simulink model "PMSM_model"  (R2014b)
settings: Solver=ode45  StartTime=0.0  StopTime=10.0  RelTol=1e-3
settings Model: CovSFcnEnable=on  Creator=Lei  LastModifiedBy=Lei
settings DataIOCC: SignalLoggingSaveFormat=ModelDataLogs  SignalLoggingName=sigsOut
settings DebuggingCC: SaveWithParameterizedLinksMsg=none  UnderspecifiedInitializationDetection=Classic  MergeDetectMultiDrivingBlocksExec=none  SignalResolutionControl=TryResolveAllWithWarning  SolverPrmCheckMsg=none  MultiTaskDSMMsg=warning  MultiTaskCondExecSysMsg=none  FrameProcessingCompatibilityMsg=error  StrictBusMsg=None
settings HardwareCC: TargetUnknown=on
settings GRTTargetCC: CombineOutputUpdateFcns=off  GRTInterface=on

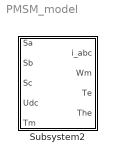
== system PMSM_model ==
  Subsystem2 : Subsystem

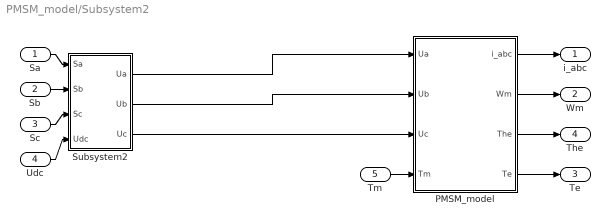
== system PMSM_model/Subsystem2 ==
  Sa : Inport
  Sb : Inport  Port=2
  Sc : Inport  Port=3
  Udc : Inport  Port=4
  Tm : Inport  Port=5
  PMSM_model : Subsystem  mask{Ld=0, Lq=0, R=0, Pn=0, flux=0, B=0, J=0}
      mask prompts: Ld "d-Inductances(Ld)"; Lq "q-Inductances(Lq)"; R "resistance(R)"; Pn "pole pairs(Pn)"; flux "Flux linkage(flux)"; B "viscous damping(B)"; J "Inertia(J)"
  Subsystem2 : Subsystem
  i_abc : Outport
  Wm : Outport  Port=2
  Te : Outport  Port=3
  The : Outport  Port=4
  wires:
  Sb/1 -> Subsystem2/2(Sb)
  Sc/1 -> Subsystem2/3(Sc)
  Udc/1 -> Subsystem2/4(Udc)
  Sa/1 -> Subsystem2/1(Sa)
  Subsystem2/1(Ua) -> PMSM_model/1(Ua)
  Subsystem2/2(Ub) -> PMSM_model/2(Ub)
  Subsystem2/3(Uc) -> PMSM_model/3(Uc)
  Tm/1 -> PMSM_model/4(Tm)
  PMSM_model/1(i_abc) -> i_abc/1
  PMSM_model/2(Wm) -> Wm/1
  PMSM_model/4(Te) -> Te/1
  PMSM_model/3(The) -> The/1

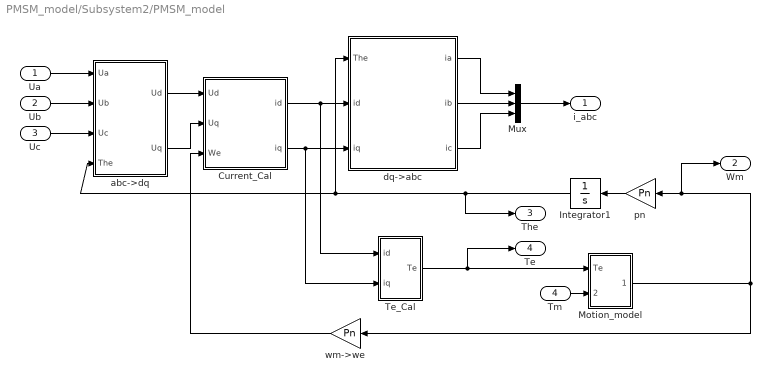
== system PMSM_model/Subsystem2/PMSM_model ==
  Ua : Inport
  Ub : Inport  Port=2
  Uc : Inport  Port=3
  Tm : Inport  Port=4
  Current_Cal : Subsystem
  Integrator1 : Integrator
  Motion_model : Subsystem
  Mux : Mux  Inputs=3
  Te_Cal : Subsystem
  abc->dq : Subsystem
  dq->abc : Subsystem
  pn : Gain  Gain=Pn  SaturateOnIntegerOverflow=on  OutDataTypeStr=Inherit: Same as input  ParamDataTypeStr=Inherit: Same as input
  wm->we : Gain  Gain=Pn  SaturateOnIntegerOverflow=on  OutDataTypeStr=Inherit: Same as input  ParamDataTypeStr=Inherit: Same as input
  i_abc : Outport
  Wm : Outport  Port=2
  The : Outport  Port=3
  Te : Outport  Port=4
  wires:
  Ua/1 -> abc->dq/1(Ua)
  abc->dq/1(Ud) -> Current_Cal/1(Ud)
  abc->dq/2(Uq) -> Current_Cal/2(Uq)
  Current_Cal/1(id) -> Te_Cal/1(id), dq->abc/2(id)
  Current_Cal/2(iq) -> Te_Cal/2(iq), dq->abc/3(iq)
  Integrator1/1 -> abc->dq/4(The), dq->abc/1(The), The/1
  dq->abc/1(ia) -> Mux/1
  pn/1 -> Integrator1/1
  Uc/1 -> abc->dq/3(Uc)
  Ub/1 -> abc->dq/2(Ub)
  dq->abc/3(ic) -> Mux/3
  Mux/1 -> i_abc/1
  dq->abc/2(ib) -> Mux/2
  wm->we/1 -> Current_Cal/3(We)
  Motion_model/1(wm) -> wm->we/1, Wm/1, pn/1
  Te_Cal/1(Te) -> Te/1, Motion_model/1(Te)
  Tm/1 -> Motion_model/2(Tm)

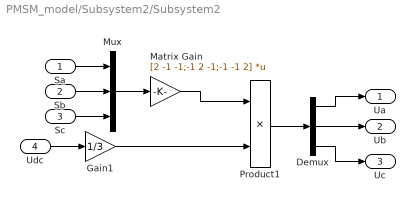
== system PMSM_model/Subsystem2/Subsystem2 ==
  Sa : Inport
  Sb : Inport  Port=2
  Sc : Inport  Port=3
  Udc : Inport  Port=4
  Demux : Demux  Outputs=3
  Gain1 : Gain  Gain=1/3  SaturateOnIntegerOverflow=on  OutDataTypeStr=Inherit: Same as input  ParamDataTypeStr=Inherit: Same as input
  Matrix Gain : Gain  Gain=[2 -1 -1;-1 2 -1;-1 -1 2]  Multiplication=Matrix(K*u)  SaturateOnIntegerOverflow=on  OutDataTypeStr=Inherit: Same as input  ParamDataTypeStr=Inherit: Same as input
  Mux : Mux  Inputs=3
  Product1 : Product  SaturateOnIntegerOverflow=on  OutDataTypeStr=Inherit: Same as first input
  Ua : Outport
  Ub : Outport  Port=2
  Uc : Outport  Port=3
  wires:
  Mux/1 -> Matrix Gain/1
  Matrix Gain/1 -> Product1/1
  Gain1/1 -> Product1/2
  Product1/1 -> Demux/1
  Demux/1 -> Ua/1
  Demux/2 -> Ub/1
  Demux/3 -> Uc/1
  Sa/1 -> Mux/1
  Sb/1 -> Mux/2
  Sc/1 -> Mux/3
  Udc/1 -> Gain1/1

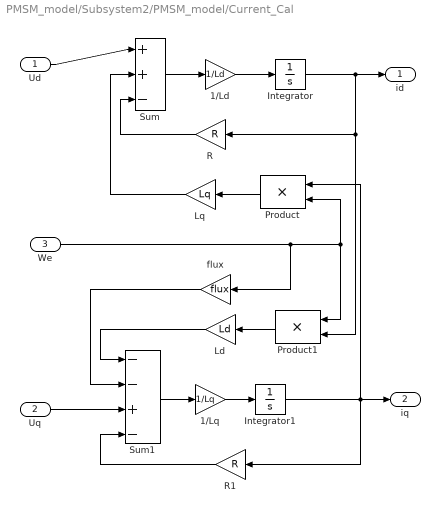
== system PMSM_model/Subsystem2/PMSM_model/Current_Cal ==
  Ud : Inport
  Uq : Inport  Port=2
  We : Inport  Port=3
  1/Ld : Gain  Gain=1/Ld  SaturateOnIntegerOverflow=on  OutDataTypeStr=Inherit: Same as input  ParamDataTypeStr=Inherit: Same as input
  1/Lq : Gain  Gain=1/Lq  SaturateOnIntegerOverflow=on  OutDataTypeStr=Inherit: Same as input  ParamDataTypeStr=Inherit: Same as input
  Integrator : Integrator  InitialCondition=0.01
  Integrator1 : Integrator
  Ld : Gain  Gain=Ld  SaturateOnIntegerOverflow=on  OutDataTypeStr=Inherit: Same as input  ParamDataTypeStr=Inherit: Same as input
  Lq : Gain  Gain=Lq  SaturateOnIntegerOverflow=on  OutDataTypeStr=Inherit: Same as input  ParamDataTypeStr=Inherit: Same as input
  Product : Product  SaturateOnIntegerOverflow=on  OutDataTypeStr=Inherit: Same as first input
  Product1 : Product  SaturateOnIntegerOverflow=on  OutDataTypeStr=Inherit: Same as first input
  R : Gain  Gain=R  SaturateOnIntegerOverflow=on  OutDataTypeStr=Inherit: Same as input  ParamDataTypeStr=Inherit: Same as input
  R1 : Gain  Gain=R  SaturateOnIntegerOverflow=on  OutDataTypeStr=Inherit: Same as input  ParamDataTypeStr=Inherit: Same as input
  Sum : Sum  Inputs=|++-  SaturateOnIntegerOverflow=on
  Sum1 : Sum  Inputs=--+-  SaturateOnIntegerOverflow=on
  flux : Gain  Gain=flux  SaturateOnIntegerOverflow=on  OutDataTypeStr=Inherit: Same as input  ParamDataTypeStr=Inherit: Same as input
  id : Outport
  iq : Outport  Port=2
  wires:
  Ud/1 -> Sum/1
  Sum/1 -> 1/Ld/1
  1/Ld/1 -> Integrator/1
  Integrator/1 -> Product1/2, R/1, id/1
  Product/1 -> Lq/1
  Lq/1 -> Sum/2
  We/1 -> Product/2, Product1/1, flux/1
  R/1 -> Sum/3
  R1/1 -> Sum1/4
  1/Lq/1 -> Integrator1/1
  Sum1/1 -> 1/Lq/1
  Integrator1/1 -> R1/1, Product/1, iq/1
  Product1/1 -> Ld/1
  Ld/1 -> Sum1/1
  Uq/1 -> Sum1/3
  flux/1 -> Sum1/2

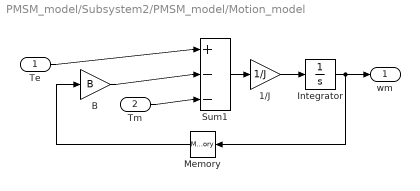
== system PMSM_model/Subsystem2/PMSM_model/Motion_model ==
  Te : Inport
  Tm : Inport  Port=2
  1/J : Gain  Gain=1/J  SaturateOnIntegerOverflow=on  OutDataTypeStr=Inherit: Same as input  ParamDataTypeStr=Inherit: Same as input
  B : Gain  Gain=B  SaturateOnIntegerOverflow=on  OutDataTypeStr=Inherit: Same as input  ParamDataTypeStr=Inherit: Same as input
  Integrator : Integrator
  Memory : Memory
  Sum1 : Sum  Inputs=|+--  SaturateOnIntegerOverflow=on
  wm : Outport
  wires:
  Tm/1 -> Sum1/3
  Sum1/1 -> 1/J/1
  B/1 -> Sum1/2
  1/J/1 -> Integrator/1
  Te/1 -> Sum1/1
  Integrator/1 -> Memory/1, wm/1
  Memory/1 -> B/1

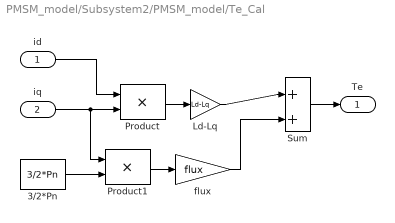
== system PMSM_model/Subsystem2/PMSM_model/Te_Cal ==
  id : Inport
  iq : Inport  Port=2
  3/2*Pn : Constant  Value=3/2*Pn
  Ld-Lq : Gain  Gain=Ld-Lq  SaturateOnIntegerOverflow=on  OutDataTypeStr=Inherit: Same as input  ParamDataTypeStr=Inherit: Same as input
  Product : Product  SaturateOnIntegerOverflow=on  OutDataTypeStr=Inherit: Same as first input
  Product1 : Product  SaturateOnIntegerOverflow=on  OutDataTypeStr=Inherit: Same as first input
  Sum : Sum  Inputs=|++  SaturateOnIntegerOverflow=on
  flux : Gain  Gain=flux  SaturateOnIntegerOverflow=on  OutDataTypeStr=Inherit: Same as input  ParamDataTypeStr=Inherit: Same as input
  Te : Outport
  wires:
  iq/1 -> Product/2, Product1/1
  id/1 -> Product/1
  3/2*Pn/1 -> Product1/2
  Ld-Lq/1 -> Sum/1
  Product/1 -> Ld-Lq/1
  flux/1 -> Sum/2
  Product1/1 -> flux/1
  Sum/1 -> Te/1

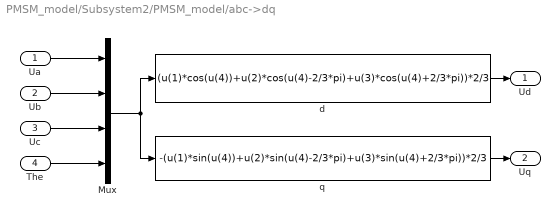
== system PMSM_model/Subsystem2/PMSM_model/abc->dq ==
  Ua : Inport
  Ub : Inport  Port=2
  Uc : Inport  Port=3
  The : Inport  Port=4
  Mux : Mux
  d : Fcn  Expr=(u(1)*cos(u(4))+u(2)*cos(u(4)-2/3*pi)+u(3)*cos(u(4)+2/3*pi))*2/3
  q : Fcn  Expr=-(u(1)*sin(u(4))+u(2)*sin(u(4)-2/3*pi)+u(3)*sin(u(4)+2/3*pi))*2/3
  Ud : Outport
  Uq : Outport  Port=2
  wires:
  Mux/1 -> q/1, d/1
  Ua/1 -> Mux/1
  Ub/1 -> Mux/2
  d/1 -> Ud/1
  The/1 -> Mux/4
  Uc/1 -> Mux/3
  q/1 -> Uq/1

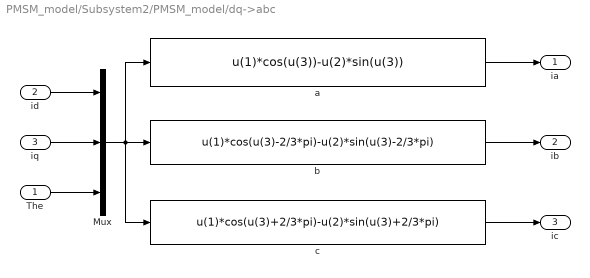
== system PMSM_model/Subsystem2/PMSM_model/dq->abc ==
  The : Inport
  id : Inport  Port=2
  iq : Inport  Port=3
  Mux : Mux  Inputs=3
  a : Fcn  Expr=u(1)*cos(u(3))-u(2)*sin(u(3))
  b : Fcn  Expr=u(1)*cos(u(3)-2/3*pi)-u(2)*sin(u(3)-2/3*pi)
  c : Fcn  Expr=u(1)*cos(u(3)+2/3*pi)-u(2)*sin(u(3)+2/3*pi)
  ia : Outport
  ib : Outport  Port=2
  ic : Outport  Port=3
  wires:
  b/1 -> ib/1
  The/1 -> Mux/3
  a/1 -> ia/1
  id/1 -> Mux/1
  iq/1 -> Mux/2
  Mux/1 -> c/1, a/1, b/1
  c/1 -> ic/1
